simulink model "LPVMPC_AGV_simulink"  (R2024b)
settings: Solver=ode4  StartTime=0.0  StopTime=20  FixedStep=0.05  RelTol=1e-3
PreLoadFcn:
  | %% PreLoadFcn - 自动路径兼容版 V3.0 (2025-12-10)
  | fprintf('\n');
  | fprintf('╔════════════════════════════════════════════════════════════╗\n');
  | fprintf('║     LPVMPC_AGV 模型初始化 (PreLoadFcn, V3.0, 2025-12-10)   ║\n');
  | fprintf('╚════════════════════════════════════════════════════════════╝\n\n');
  | 
  | %% Bootstrap path + 目录配置
  | init_project();
  | root = project_root();
  | data_dir = fullfile(root, 'data');
  | data_models_dir = fullfile(data_dir, 'models');
  | data_paths_dir = fullfile(data_dir, 'paths');
  | data_gru_dir = fullfile(data_dir, 'gru');
  | results_root = results_dir('');
  | results_paths = struct( ...
  |     'root', results_root, ...
  |     'simulink', results_dir('simulink'), ...
  |     'closed_loop', results_dir('closed_loop'), ...
  |     'paths', results_dir('paths'), ...
  |     'gru_logs', results_dir('gru/sim'));
  | env_paths = struct('root', root, 'data', data_dir, 'models', data_models_dir, ...
  |     'paths', data_paths_dir, 'gru', data_gru_dir, 'results', results_paths);
  | 
  | assignin('base', 'results_paths', results_paths);
  | assignin('base', 'env_paths', env_paths);
  | 
  | mw = get_param(bdroot, 'ModelWorkspace');
  | assignin(mw, 'results_paths', results_paths);
  | assignin(mw, 'env_paths', env_paths);
  | try, save(mw); catch, end
  | 
  | %% 步骤0：加载基础参数
  | fprintf('[步骤 0/6] 加载基础参数...\n');
  | try
  |     params = parameters();
  |     fprintf('  ✓ parameters() 加载成功 (Ts=%.3fs, m=%.1fkg, L=%.2fm)\n', ...
  |         params.Ts, params.mass, params.L);
  | catch ME
  |     warning('[PreLoadFcn] parameters() 失败: %s', ME.message);
  |     params = struct('Ts',0.05,'mass',100,'gravity',9.81, ...
  |         'rolling_resistance',0.015,'air_density',1.225, ...
  |         'drag_coefficient_area',0.5,'L',2.0);
  | end
  | assignin('base','params',params);
  | assignin(mw,'params',params);
  | 
  | ff_rt = struct('m',params.mass,'g',params.gravity, ...
  |     'c_r',params.rolling_resistance,'rho',params.air_density, ...
  |     'CdA',params.drag_coefficient_area);
  | v_ff_nom = 1.0;
  | assignin('base','ff_rt',ff_rt);
  | assignin('base','v_ff_nom',v_ff_nom);
  | assignin(mw,'ff_rt',ff_rt);
  | assignin(mw,'v_ff_nom',v_ff_nom);
  | try, save(mw); catch, end
  | fprintf('\n');
  | 
  | %% 步骤1：载入 LPV 数据库
  | fprintf('[步骤 1/6] 加载 LPV 数据库...\n');
  | base_names = {'lin_agv_db.mat','plant_grid_test.mat','plant_grid.mat'};
  | base_dirs = {data_models_dir, root, ''};
  | db_files = {};
  | for d = 1:numel(base_dirs)
  |     for n = 1:numel(base_names)
  |         if isempty(base_dirs{d})
  |             db_files{end+1} = base_names{n}; %#ok<AGROW>
  |         else
  |             db_files{end+1} = fullfile(base_dirs{d}, base_names{n}); %#ok<AGROW>
  |         end
  |     end
  | end
  | db_files = unique(db_files, 'stable');
  | 
  | S = [];
  | loaded_db_file = '';
  | for i = 1:numel(db_files)
  |     if exist(db_files{i}, 'file')
  |         try
  |             S = load(db_files{i});
  |             loaded_db_file = db_files{i};
  |             fprintf('  ✓ 文件加载成功: %s\n', db_files{i});
  |             break;
  |         catch ME
  |             fprintf('  ⚠ 尝试加载 %s 失败: %s\n', db_files{i}, ME.message);
  |         end
  |     end
  | end
  | 
  | if isempty(S)
  |     error('[PreLoadFcn] ❌ 未找到 LPV 数据库文件（请先运行 lin_agv_grid 或 test_lpvmpc_workflow）');
  | end
  | 
  | if isfield(S,'db') && isstruct(S.db)
  |     db_data = S.db;
  |     fprintf('  → 使用 db 结构体格式\n');
  | elseif all(isfield(S, {'A','B','C','D','E'}))
  |     db_data = S;
  |     fprintf('  → 使用顶层字段格式\n');
  | else
  |     error('[PreLoadFcn] 数据库格式无法识别 (字段: %s)', strjoin(fieldnames(S), ', '));
  | end
  | 
  | req = {'A','B','C','D','E','Ts','grid'};
  | missing = req(~isfield(db_data, req));
  | if ~isempty(missing)
  |     error('[PreLoadFcn] ❌ 数据库缺少字段: %s', strjoin(missing, ', '));
  | end
  | 
  | A=db_data.A; B=db_data.B; C=db_data.C; D=db_data.D; E=db_data.E;
  | Ts=db_data.Ts; grid=db_data.grid;
  | nx=size(A,4); nu=size(B,5); ny=size(C,4); nd=size(E,5);
  | Nv=size(A,1); Nw=size(A,2); Nt=size(A,3);
  | 
  | fprintf('  ✓ 网格: %d×%d×%d (总 %d 点), nx=%d, nu=%d, nd=%d, Ts=%.3fs\n', ...
  |     Nv, Nw, Nt, Nv*Nw*Nt, nx, nu, nd, Ts);
  | 
  | db_rt = struct('A',A,'B',B,'C',C,'D',D,'E',E, ...
  |     'grid',grid,'Ts',Ts,'nx',nx,'nu',nu,'ny',ny,'nd',nd, ...
  |     'Nv',Nv,'Nw',Nw,'Nt',Nt);
  | assignin('base','db_rt',db_rt);
  | assignin(mw,'db_rt',db_rt);
  | try, save(mw); catch, end
  | fprintf('\n');
  | 
  | %% 步骤2：创建 MPCPlantBus
  | fprintf('[步骤 2/6] 创建 MPCPlantBus...\n');
  | nu_md = nu + nd;
  | samplePlant = struct('A',zeros(nx,nx),'B',zeros(nx,nu_md), ...
  |     'C',zeros(ny,nx),'D',zeros(ny,nu_md),'U',zeros(nu_md,1), ...
  |     'X',zeros(nx,1),'Y',zeros(ny,1),'DX',zeros(nx,1),'Ts',Ts);
  | info = Simulink.Bus.createObject(samplePlant);
  | assignin('base','MPCPlantBus', eval(info.busName));
  | if ~strcmp(info.busName,'MPCPlantBus')
  |     eval(sprintf('clear %s;', info.busName));
  | end
  | assignin('base','plant_ic', samplePlant);
  | fprintf('  ✓ MPCPlantBus 创建成功 (nu_md=%d = %d MV + %d MD)\n\n', nu_md, nu, nd);
  | 
  | %% 步骤3：加载 maps_best / ctrl
  | fprintf('[步骤 3/6] 加载 maps_best / ctrl...\n');
  | base_dirs_mb = {data_models_dir, root, ''};
  | maps_files = {};
  | for d = 1:numel(base_dirs_mb)
  |     if isempty(base_dirs_mb{d})
  |         maps_files{end+1} = 'maps_best.mat'; %#ok<AGROW>
  |     else
  |         maps_files{end+1} = fullfile(base_dirs_mb{d}, 'maps_best.mat'); %#ok<AGROW>
  |     end
  | end
  | maps_files = unique(maps_files, 'stable');
  | 
  | maps_best = [];
  | maps_loaded = false;
  | for i = 1:numel(maps_files)
  |     if exist(maps_files{i}, 'file')
  |         try
  |             Tm = load(maps_files{i});
  |             if isfield(Tm,'maps_best')
  |                 maps_best = Tm.maps_best;
  |                 maps_loaded = true;
  |                 fprintf('  ✓ maps_best 加载成功 (%s)\n', maps_files{i});
  |                 if isfield(maps_best,'version')
  |                     fprintf('    - 版本: %s\n', maps_best.version);
  |                 end
  |                 if isfield(maps_best,'timestamp')
  |                     fprintf('    - 时间: %s\n', maps_best.timestamp);
  |                 end
  |             end
  |             break;
  |         catch ME
  |             fprintf('  ⚠ 加载 %s 失败: %s\n', maps_files{i}, ME.message);
  |         end
  |     end
  | end
  | if ~maps_loaded
  |     fprintf('  ⚠ 未找到 maps_best.mat，使用默认权重\n');
  | end
  | 
  | ctrl = [];
  | ctrl_source = '未创建';
  | base_dirs_ctrl = {data_models_dir, root};
  | ctrl_files = {};
  | for d = 1:numel(base_dirs_ctrl)
  |     ctrl_files{end+1} = fullfile(base_dirs_ctrl{d}, 'ctrl.mat'); %#ok<AGROW>
  | end
  | ctrl_files = unique(ctrl_files, 'stable');
  | 
  | for i = 1:numel(ctrl_files)
  |     if exist(ctrl_files{i}, 'file')
  |         try
  |             Tc = load(ctrl_files{i});
  |             if isfield(Tc,'ctrl')
  |                 ctrl = Tc.ctrl;
  |                 ctrl_source = ctrl_files{i};
  |                 fprintf('  ✓ 从 %s 加载 ctrl\n', ctrl_source);
  |                 break;
  |             end
  |         catch ME
  |             fprintf('  ⚠ 加载 %s 失败: %s\n', ctrl_files{i}, ME.message);
  |         end
  |     end
  | end
  | 
  | if isempty(ctrl) && exist('mpc_setup_single_interp','file')==2
  |     fprintf('  → 创建新控制器...\n');
  |     if maps_loaded && all(isfield(maps_best, {'Q_range','R_range','dR_range'}))
  |         Q_base = mean(maps_best.Q_range,1);
  |         R_base = mean(maps_best.R_range,1);
  |         dR_base = mean(maps_best.dR_range,1);
  |         fprintf('    使用 maps_best 权重\n');
  |     else
  |         Q_base = [3,8,1,1];
  |         R_base = [1e-3,1e-3];
  |         dR_base = [1e-2,1e-2];
  |         fprintf('    使用默认权重\n');
  |     end
  |     mpc_opts = struct('Np',30,'Nc',10,'Q',Q_base,'R',R_base,'dR',dR_base);
  |     ctrl = mpc_setup_single_interp(db_rt, mpc_opts);
  |     ctrl_source = '新创建';
  |     fprintf('  ✓ 控制器创建成功 (P=%.2fs, M=%.2fs)\n', ...
  |         ctrl.meta.prediction_horizon_sec, ctrl.meta.control_horizon_sec);
  | end
  | 
  | if maps_loaded && ~isempty(ctrl)
  |     fields = {'Q_range','R_range','dR_range','alpha_Q','beta_Q', ...
  |         'alpha_R','beta_R','alpha_dR','beta_dR', ...
  |         'scale_umin_lo','scale_umin_hi','scale_umax_lo','scale_umax_hi'};
  |     copied = 0;
  |     for i = 1:numel(fields)
  |         if isfield(maps_best, fields{i})
  |             ctrl.maps.(fields{i}) = maps_best.(fields{i});
  |             copied = copied + 1;
  |         end
  |     end
  |     fprintf('  → 已将 %d 个 maps_best 字段写入 ctrl.maps\n', copied);
  | end
  | 
  | if ~isempty(ctrl)
  |     assignin('base','ctrl',ctrl);
  | else
  |     warning('[PreLoadFcn] 无法创建/加载 ctrl');
  | end
  | fprintf('\n');
  | 
  | %% 步骤4：直接加载参考路径到基础工作区
  | % fprintf('[步骤 4/6] 加载路径参考数据（ref_* 格式）...\n');
  | %
  | % path_types = {'straight','turn','straight_left_turn','straight_right_turn','slope','bumpy', ...
  | %               's_curve','s_shape'};
  | % path_refs = struct();
  | % paths_loaded = 0;
  | %
  | % for i = 1:numel(path_types)
  | %     name = path_types{i};
  | %     file_path = fullfile(data_paths_dir, sprintf('path_%s.mat', name));
  | %     if ~exist(file_path,'file')
  | %         fprintf('  ⚠ 缺少路径文件: %s\n', file_path);
  | %         continue;
  | %     end
  | %
  | %     try
  | %         data = load(file_path);
  | %         if ~isfield(data,'ref')
  | %             error('文件缺少 ref 结构');
  | %         end
  | %         ref = data.ref;
  | %         var_name = sprintf('ref_%s', name);
  | %
  | %         % 写入 Base Workspace（兼容旧流程）
  | %         assignin('base', var_name, ref);
  | %         % 如需模型工作区可同步写入
  | %         assignin(mw, var_name, ref);
  | %
  | %         % 记录到 path_refs 结构
  | %         path_refs.(name) = ref;
  | %
  | %         paths_loaded = paths_loaded + 1;
  | %         fprintf('  ✓ %s: 已加载 (%s → %s)\n', name, file_path, var_name);
  | %     catch ME
  | %         fprintf('  ❌ 加载 %s 失败: %s\n', name, ME.message);
  | %     end
  | % end
  | %
  | % assignin('base','path_refs',path_refs);
  | % assignin(mw,'path_refs',path_refs);
  | % try, save(mw); catch, end
  | % fprintf('  → 路径数据加载 %d/%d\n\n', paths_loaded, numel(path_types));
  | %% 步骤5：加载 GRU 模型
  | fprintf('[步骤 5/6] 加载 GRU 模型...\n');
  | gru_model = [];
  | gru_scaler = [];
  | 
  | base_dirs_gru = {data_models_dir, data_gru_dir, root};
  | gru_files = {};
  | for d = 1:numel(base_dirs_gru)
  |     gru_files{end+1} = fullfile(base_dirs_gru{d}, 'GRU_model.mat'); %#ok<AGROW>
  | end
  | gru_files = unique(gru_files, 'stable');
  | 
  | for i = 1:numel(gru_files)
  |     if exist(gru_files{i},'file')
  |         Sg = load(gru_files{i});
  |         if isfield(Sg,'model')
  |             gru_model = Sg.model;
  |             fprintf('  ✓ GRU_model 加载成功 (%s)\n', gru_files{i});
  |             if isfield(gru_model,'seq_len')
  |                 fprintf('    - 序列长度: %d\n', gru_model.seq_len);
  |             end
  |             if isfield(gru_model,'scaler')
  |                 gru_scaler = gru_model.scaler;
  |             end
  |             break;
  |         end
  |     end
  | end
  | if isempty(gru_model)
  |     error('[PreLoadFcn] ❌ 未找到 GRU_model.mat');
  | end
  | 
  | scaler_files = {};
  | for d = 1:numel(base_dirs_gru)
  |     scaler_files{end+1} = fullfile(base_dirs_gru{d}, 'GRU_scaler.mat'); %#ok<AGROW>
  | end
  | scaler_files = unique(scaler_files, 'stable');
  | if isempty(gru_scaler)
  |     for i = 1:numel(scaler_files)
  |         if exist(scaler_files{i},'file')
  |             Ss = load(scaler_files{i});
  |             if isfield(Ss,'scaler')
  |                 gru_scaler = Ss.scaler;
  |                 fprintf('  ✓ GRU_scaler 加载成功 (%s)\n', scaler_files{i});
  |                 break;
  |             end
  |         end
  |     end
  | end
  | 
  | assignin('base','gru_model',gru_model);
  | if ~isempty(gru_scaler)
  |     assignin('base','gru_scaler',gru_scaler);
  | end
  | fprintf('\n');
  | 
  | %% 步骤6：总结
  | fprintf('[步骤 6/6] 初始化总结\n');
  | fprintf('  ════════════════════════════════════════════════\n');
  | fprintf('  ✓ 基础参数:     已加载\n');
  | fprintf('  ✓ LPV 数据库:   %s (%d×%d×%d)\n', loaded_db_file, Nv, Nw, Nt);
  | fprintf('  ✓ MPCPlantBus:  已创建\n');
  | % fprintf('  ✓ 路径数据:     %d/%d\n', paths_loaded, numel(path_types));
  | fprintf('  ✓ GRU 模型:     就绪\n');
  | if maps_loaded
  |     fprintf('  ✓ maps_best:    已加载\n');
  | else
  |     fprintf('  ⚠ maps_best:    未加载\n');
  | end
  | if ~isempty(ctrl)
  |     fprintf('  ✓ MPC 控制器:   %s\n', ctrl_source);
  | else
  |     fprintf('  ❌ MPC 控制器:  未创建\n');
  | end
  | fprintf('  ════════════════════════════════════════════════\n');
  | 
  | if maps_loaded && ~isempty(ctrl)
  |     fprintf('\n✓ 初始化成功！使用优化权重与 GRU 调度\n');
  | elseif ~isempty(ctrl)
  |     fprintf('\n⚠ 初始化完成，使用默认权重\n');
  | else
  |     fprintf('\n❌ 初始化失败，请检查上方日志\n');
  | end
  | fprintf('\n[PreLoadFcn] 完成\n\n');
model workspace (MAT data in the model file):
  CdA = 0.5
  MPC_idx = [1 2 3 4]
  c_r = 0.015
  db_rt.A = [1 1 1 1 1 1 1 1 1 1 1 1 ... (2000 elements, 5x5x5x4x4)]
  db_rt.B = [1.10696819051e-09 6.56859347141e-11 7.70788358052e-11 4.63456222969e-11 -1.91478442817e-11 3.08062125377e-10 3.17967815903e-10 3.27251111689e-10 3.36091973111e-10 3.44604983367e-10 -2.40695313568e-13 -1.34215112609e-13 ... (1000 elements, 5x5x5x4x2)]
  db_rt.C = [1 1 1 1 1 1 1 1 1 1 1 1 ... (2000 elements, 5x5x5x4x4)]
  db_rt.D = [0 0 0 0 0 0 0 0 0 0 0 0 ... (1000 elements, 5x5x5x4x2)]
  db_rt.E = [2.11033585519e-07 -6.42122832244e-08 -7.53495772598e-08 -4.53058513965e-08 1.871832239e-08 -3.01151562194e-07 -3.10835010863e-07 -3.19910021986e-07 -3.2855251907e-07 -3.36874515032e-07 2.35296065713e-10 1.31204413144e-10 ... (500 elements, 5x5x5x4)]
  db_rt.grid.V = [0.8; 0.9; 1; 1.1; 1.2]
  db_rt.grid.W = [-0.2; -0.1; 0; 0.1; 0.2]
  db_rt.grid.T = [-0.1; -0.05; 0; 0.05; 0.1]
  db_rt.Ts = 0.01
  db_rt.nx = 4
  db_rt.nu = 2
  db_rt.ny = 4
  db_rt.nd = 1
  db_rt.Nv = 5
  db_rt.Nw = 5
  db_rt.Nt = 5
  g = 9.81
  m = 100
  rho = 1.225
libraries: mpclib x1
settings Model: Creator=15754  LastModifiedBy=15754

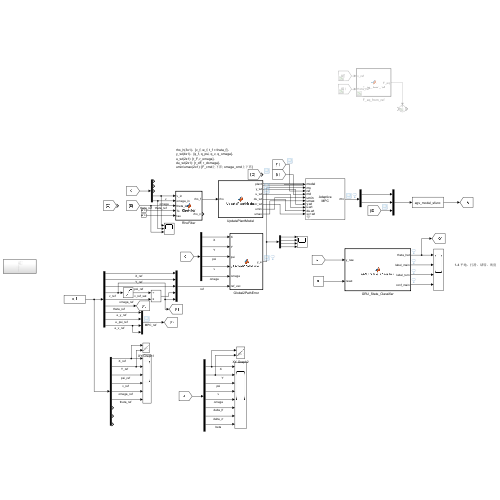
[thumbnail: Simulink's stored preview of the top-level diagram]
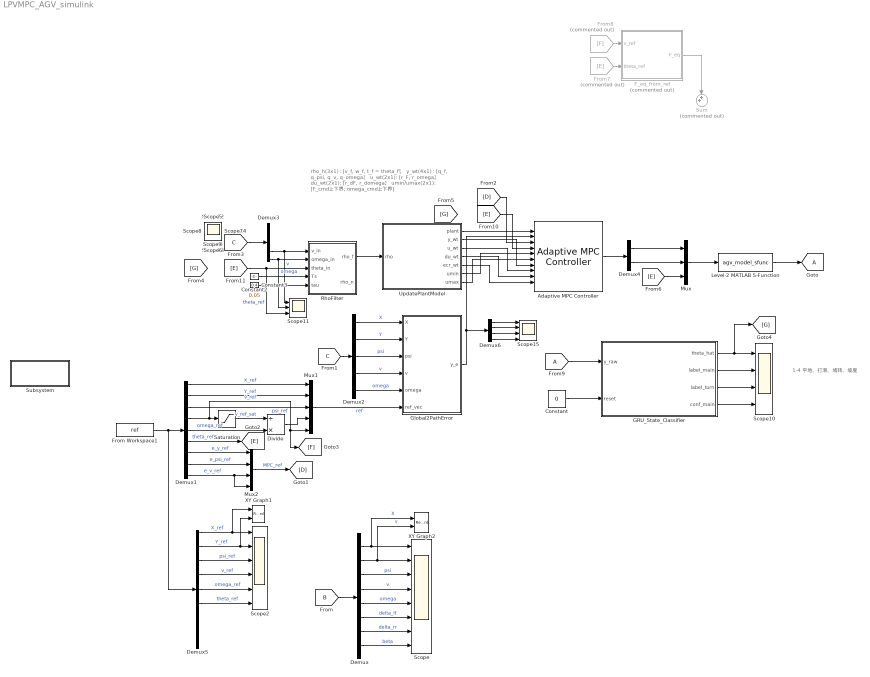
== system LPVMPC_AGV_simulink ==
  note: rho_h(3x1)：[v_f, w_f, t_f = theta_f]。
      | y_wt(4x1)：[q_f, q_psi, q_v, q_omega]。
      | u_wt(2x1): [r_F, r_omega]。
      | du_wt(2x1): [r_dF, r_domega]。
      | umin/umax(2x1): [F_cmd上下界; omega_cmd上下界]
  note: 1-4 平地、打滑、堵转、坡度
  Adaptive MPC Controller : mpclib/Adaptive MPC Controller  SCDEnableBlockLinearizationSpecification=on  mpcobj=ctrl.mpcobj  enable_value=0  updateMPCinCallerWorkspace=on  md_inport=on  mv_inport=off  uref_inport=off  return_cost=off  return_mvseq=off  return_qpstatus=off  return_xseq=off  return_state=off  return_ovseq=off  state_inport=off  isltv_plant=off  umin_inport=on  umax_inport=on  ymin_inport=off  ymax_inport=off  cc_inport=off  ywt_inport=on  uwt_inport=on  duwt_inport=on  rhoeps_inport=on  pm_inport=off  MaximumP=10  HorizonChoice=FixedHorizon  BlockDataType=double  SampleTimeInherited=off  switch_inport=off
  Constant : Constant  Value=0  SampleTime=params.Ts
  Constant2 : Constant  Value=0.05  SampleTime=params.Ts
  Constant3 : Constant  Value=0.4  SampleTime=params.Ts
  Demux : Demux  Outputs=8
  Demux1 : Demux  Outputs=9
  Demux2 : Demux  Outputs=5
  Demux3 : Demux  Outputs=5
  Demux4 : Demux  Outputs=2
  Demux5 : Demux  Outputs=9
  Demux6 : Demux
  Divide : Product  Inputs=/*
  F_eq_from_ref : MATLAB Function  Commented=on  TreatAsAtomicUnit=on
  From Workspace1 : FromWorkspace  VariableName=ref  SampleTime=0.05
  From7 : From  Commented=on  GotoTag=E
  From8 : From  Commented=on  GotoTag=F
  From9 : From  TagVisibility=global
  GRU_State_Classifier : MATLAB Function  TreatAsAtomicUnit=on
  Global2PathError : MATLAB Function  TreatAsAtomicUnit=on  SystemSampleTime=params.Ts
  Goto : Goto  TagVisibility=global
  Level-2 MATLAB S-Function : M-S-Function  FunctionName=agv_model_sfunc  Parameters=parameters
  Mux : Mux  Inputs=3
  Mux1 : Mux  Inputs=5
  Mux2 : Mux
  RhoFilter : MATLAB Function  TreatAsAtomicUnit=on  SystemSampleTime=0.05
  Saturation : Saturate  UpperLimit=Inf  LowerLimit=1e-3
  Scope : Scope  NumInputPorts=8
  Scope10 : Scope  NumInputPorts=4
  Scope11 : Scope  NumInputPorts=3
  Scope15 : Scope  NumInputPorts=4
  Scope2 : Scope  NumInputPorts=6
  Subsystem : Subsystem
  Sum : Sum  Commented=on  Inputs=++|
  UpdatePlantModel : MATLAB Function  TreatAsAtomicUnit=on
  XY Graph1 : Record  FileSettingsInternal="{\"entries\":[{\"content\":{\"excelSettings\":{\"content\":{},\"type\":\"Streamout.ExcelSettings\"}},\"type\":\"Streamout.FileSettingStorage\",\"uuid\":\"\"}],\"packageUris\":[\"http:\\/\\/schema.mathworks.com\\/mf0\\/streamout_blocks\\/R2020a\"],\"version\":\"1.0\"}"  Layout=[1 1]  SignalsInternal="{\"entries\":[{\"content\":{\"signals\":[{\"content\":{\"blockPath\":[],\"dimensions\":[1],\"domain\":\"\",\"lineColor\":\"#a2142f\",\"plots\":[ 1 ],\"port\":1,\"sid\":[\"\"],\"signalID\":1,\"signalName\":\"X_ref\"},\"type\":\"RecordBlkView.Signal\",\"uuid\":\"\"},{\"content\":{\"blockPath\":[],\"dimensions\":[1],\"domain\":\"\",\"lineColor\":\"#139fff\",\"plots\":[ 1 ],\"port\":2,\"sid\":[\"\"],\"signalID\":2,\"signalName\":\"Y_ref\"},\"type\":\"RecordBlkView.Signal\",\"uuid\":\"\"}]},\"type\":\"RecordBlkView.InputSignals\",\"uuid\":\"\"}],\"packageUris\":[\"http:\\/\\/schema.mathworks.com\\/mf0\\/streamout_blocks\\/R2020a\"],\"version\":\"1.0\"}"  VisualizationBindings="{\"xyplotplugin\":{\"info\":[{\"series\":[{\"bindingParametersList\":[{\"parameter\":\"X-Axis\",\"signalID\":1,\"signalName\":\"X_ref\"},{\"parameter\":\"Y-Axis\",\"signalID\":2,\"signalName\":\"Y_ref\"}],\"seriesID\":0}],\"subplotID\":1}]}}"  CompatibilityTag=XY
  XY Graph2 : Record  FileSettingsInternal="{\"entries\":[{\"content\":{\"excelSettings\":{\"content\":{},\"type\":\"Streamout.ExcelSettings\"}},\"type\":\"Streamout.FileSettingStorage\",\"uuid\":\"\"}],\"packageUris\":[\"http:\\/\\/schema.mathworks.com\\/mf0\\/streamout_blocks\\/R2020a\"],\"version\":\"1.0\"}"  Layout=[1 1]  SignalsInternal="{\"entries\":[{\"content\":{\"signals\":[{\"content\":{\"blockPath\":[],\"dimensions\":[1],\"domain\":\"\",\"lineColor\":\"#a2142f\",\"plots\":[ 1 ],\"port\":1,\"sid\":[\"\"],\"signalID\":1,\"signalName\":\"X\"},\"type\":\"RecordBlkView.Signal\",\"uuid\":\"\"},{\"content\":{\"blockPath\":[],\"dimensions\":[1],\"domain\":\"\",\"lineColor\":\"#139fff\",\"plots\":[ 1 ],\"port\":2,\"sid\":[\"\"],\"signalID\":2,\"signalName\":\"Y\"},\"type\":\"RecordBlkView.Signal\",\"uuid\":\"\"}]},\"type\":\"RecordBlkView.InputSignals\",\"uuid\":\"\"}],\"packageUris\":[\"http:\\/\\/schema.mathworks.com\\/mf0\\/streamout_blocks\\/R2020a\"],\"version\":\"1.0\"}"  VisualizationBindings="{\"xyplotplugin\":{\"info\":[{\"series\":[{\"bindingParametersList\":[{\"parameter\":\"X-Axis\",\"signalID\":1,\"signalName\":\"X\"},{\"parameter\":\"Y-Axis\",\"signalID\":2,\"signalName\":\"Y\"}],\"seriesID\":0}],\"subplotID\":1}]}}"  CompatibilityTag=XY
  Scope{1,3..9,12..14} (11 alike) : Scope
  wires:
  Level-2 MATLAB S-Function/1 -> Goto/1
  [B] -> Demux/1
  Demux/1 -> XY Graph2/1, Scope/1  "X"
  Demux/2 -> XY Graph2/2, Scope/2  "Y"
  Demux/3 -> Scope/3  "psi"
  Demux/4 -> Scope/4  "v"
  Demux/5 -> Scope/5  "omega"
  Demux/6 -> Scope/6  "delta_lf"
  Demux/7 -> Scope/7  "delta_rr"
  Demux/8 -> Scope/8  "beta"
  Demux1/4 -> [F], Mux1/5, Saturation/1  "v_ref"
  Saturation/1 -> Divide/1  "v_ref_sat"
  Demux1/5 -> Divide/2  "omega_ref"
  Demux1/1 -> Mux1/1  "X_ref"
  Demux1/2 -> Mux1/2  "Y_ref"
  Demux1/3 -> Mux1/3  "psi_ref"
  Divide/1 -> Mux1/4
  Mux1/1 -> Global2PathError/6(ref_vec)  "ref"
  [C] -> Demux2/1
  Demux2/3 -> Global2PathError/3(psi)  "psi"
  Demux2/4 -> Global2PathError/4(v)  "v"
  Demux2/5 -> Global2PathError/5(omega)  "omega"
  Demux2/2 -> Global2PathError/2(Y)  "Y"
  Demux2/1 -> Global2PathError/1(X)  "X"
  Demux1/8 -> Mux2/2  "e_psi_ref"
  Demux1/7 -> Mux2/1  "e_y_ref"
  Demux1/9 -> Mux2/4, Mux2/3  "e_v_ref"
  Mux2/1 -> [D]  "MPC_ref"
  [D] -> Adaptive MPC Controller/3
  [C] -> Demux3/1
  Demux3/4 -> Scope11/1, RhoFilter/1(v_in)  "v"
  Demux3/5 -> Scope11/2, RhoFilter/2(omega_in)  "omega"
  Demux1/6 -> [E]  "theta_ref"
  [E] -> Scope11/3, RhoFilter/3(theta_in)  "theta_ref"
  Constant2/1 -> RhoFilter/4(Ts)
  Constant3/1 -> RhoFilter/5(tau)
  UpdatePlantModel/1(plant) -> Adaptive MPC Controller/1
  [E] -> Adaptive MPC Controller/4
  RhoFilter/1(rho_f) -> UpdatePlantModel/1(rho)
  Demux5/1 -> XY Graph1/1, Scope2/1  "X_ref"
  Demux5/2 -> XY Graph1/2, Scope2/2  "Y_ref"
  Demux5/3 -> Scope2/3  "psi_ref"
  Demux5/4 -> Scope2/4  "v_ref"
  Demux5/5 -> Scope2/5  "omega_ref"
  Demux5/6 -> Scope2/6  "theta_ref"
  UpdatePlantModel/6(umin) -> Adaptive MPC Controller/5
  UpdatePlantModel/7(umax) -> Adaptive MPC Controller/6
  UpdatePlantModel/2(y_wt) -> Adaptive MPC Controller/7
  UpdatePlantModel/3(u_wt) -> Adaptive MPC Controller/8
  UpdatePlantModel/4(du_wt) -> Adaptive MPC Controller/9
  UpdatePlantModel/5(ecr_wt) -> Adaptive MPC Controller/10
  Global2PathError/1(y_e) -> Demux6/1, Adaptive MPC Controller/2
  Mux/1 -> Level-2 MATLAB S-Function/1
  Adaptive MPC Controller/1 -> Demux4/1
  [E] -> Mux/3
  Demux4/2 -> Mux/2
  F_eq_from_ref/1(F_eq) -> Sum/1
  From8/1 -> F_eq_from_ref/1(v_ref)
  From7/1 -> F_eq_from_ref/2(theta_ref)
  Demux4/1 -> Mux/1
  From9/1 -> GRU_State_Classifier/1(y_raw)
  GRU_State_Classifier/4(conf_main) -> Scope10/4
  GRU_State_Classifier/2(label_main) -> Scope10/2
  Constant/1 -> GRU_State_Classifier/2(reset)
  GRU_State_Classifier/3(label_turn) -> Scope10/3
  GRU_State_Classifier/1(theta_hat) -> [G], Scope10/1
  From Workspace1/1 -> Demux5/1, Demux1/1
  Demux6/1 -> Scope15/1
  Demux6/2 -> Scope15/2
  Demux6/3 -> Scope15/3
  Demux6/4 -> Scope15/4

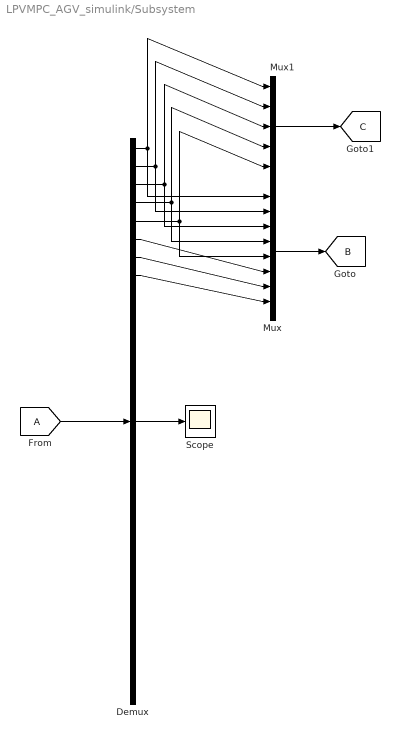
== system LPVMPC_AGV_simulink/Subsystem ==
  Demux : Demux  Outputs=31
  From : From  TagVisibility=global
  Mux : Mux  Inputs=8
  Mux1 : Mux  Inputs=5
  Scope : Scope
  tag scope: B=global, C=global
  wires:
  From/1 -> Demux/1
  Demux/1 -> Mux1/1, Mux/1
  Demux/2 -> Mux1/2, Mux/2
  Demux/3 -> Mux1/3, Mux/3
  Demux/4 -> Mux1/4, Mux/4
  Demux/5 -> Mux1/5, Mux/5
  Demux/6 -> Mux/6
  Demux/7 -> Mux/7
  Demux/8 -> Mux/8
  Mux/1 -> [B]
  Mux1/1 -> [C]
  Demux/16 -> Scope/1

== matlab function LPVMPC_AGV_simulink/RhoFilter ==
  data: v_in input; rho_f output; omega_in input; theta_in input; Ts input; tau input; rho_n output
function [rho_f, rho_n] = RhoFilter(v_in, omega_in, theta_in, Ts, tau)
% 一阶离散滤波
persistent v_f_prev w_f_prev t_f_prev
if isempty(v_f_prev), v_f_prev = 0; end
if isempty(w_f_prev), w_f_prev = 0; end
if isempty(t_f_prev), t_f_prev = 0; end

a = Ts / max(tau + Ts, 1e-6);

v_f = (1 - a)*v_f_prev + a*max(v_in, 0);   % 速度不取负·
w_f = (1 - a)*w_f_prev + a*omega_in;       % 保留符号
t_f = (1 - a)*t_f_prev + a*theta_in;       % 保留符号

v_f_prev = v_f; w_f_prev = w_f; t_f_prev = t_f;

rho_f = [v_f; w_f; t_f];

% 可选归一化（仅用于监控/调试，不参与UpdatePlantModel）
Vmax = 2.0; Wmax = 0.8; Tmax = deg2rad(10);
rho_n = [min(v_f/Vmax,1); min(abs(w_f)/Wmax,1); min(abs(t_f)/Tmax,1)];
end

== matlab function LPVMPC_AGV_simulink/Global2PathError ==
  data: X input; y_e output; Y input; psi input; v input; omega input; ref_vec input
% 误差计算模块
function y_e = Global2PathError(X, Y, psi, v, omega, ref_vec)
% ref_vec = [X_ref; Y_ref; psi_ref; kappa_ref; v_ref]
% 输出: y_e = [e_y; e_psi; e_v; e_omega; e_s]

%#codegen
% 1) 解包参考
Xr = ref_vec(1);
Yr = ref_vec(2);
psir = ref_vec(3);
kappa = ref_vec(4);
v_ref = ref_vec(5);

% 2) 横向误差：沿参考法向量投影（带符号）
ex = X - Xr; 
ey = Y - Yr;
e_y = -sin(psir)*ex + cos(psir)*ey;

% 3) 航向、速度、角速度误差
e_psi   = wrapToPi(psi - psir);
e_v     = v - v_ref;
omega_ff= v_ref * kappa;           % 曲率前馈
e_omega = omega - omega_ff;

% 4) 进度误差（可选，如未使用可置 0）
e_s = 0;

y_e = [e_y; e_psi; e_v; e_omega];
end

== matlab function LPVMPC_AGV_simulink/UpdatePlantModel ==
  data: rho input; plant output Bus: MPCPlantBus; db_rt parameter; MPC_idx parameter double size=[1 4]; ff_rt parameter; v_ff_nom parameter; y_wt output; u_wt output; du_wt output; ecr_wt output; umin output; umax output
function [plant, y_wt, u_wt, du_wt, ecr_wt, umin, umax] = UpdatePlantModel(rho, db_rt, MPC_idx, ff_rt, v_ff_nom)
%#codegen

% 标称权重/约束
Q0  = [16.3225, 29.0359, 6.9898, 2.7642];
% Q0  = [3, 8, 1, 1];
R0  = [1e-3, 1e-3];
dR0 = [1e-2, 1e-2];
umin0 = [-300; -0.6];
umax0 = [ 300;  0.6];

% 纯数值 maps：启用 ρ→(Q/R/dR/umin/umax)
maps_local = struct();
maps_local.enable_weight_interp = true;
maps_local.Q_range  = [0.5*Q0; 1.5*Q0];
maps_local.R_range  = [0.5*R0; 1.5*R0];
maps_local.dR_range = [0.5*dR0; 1.5*dR0];
% 约束：随 |ω| 插值（行1→行2）
maps_local.umin_range = [ (1.20*umin0).'; (1.00*umin0).' ];
maps_local.umax_range = [ (1.00*umax0).'; (1.20*umax0).' ];

% 在线插值
upd = mpc_update_from_rho(rho, db_rt, maps_local);

% 组装 3 输入（2 MV + 1 MD）
A   = upd.A; Bmv = upd.B; C = upd.C; Dmv = upd.D;
nx  = size(A,1); ny = size(C,1); nd = 1;
if isfield(upd,'E') && ~isempty(upd.E), Bmd = upd.E(:,1); else, Bmd = zeros(nx,1); end
Dmd = zeros(ny,nd);

plant.A = A;
plant.B = [Bmv, Bmd];   % 4x3
plant.C = C;
plant.D = [Dmv, Dmd];   % 4x3

% 名义 U（仅滚阻+风阻；坡度由 MD 处理）
% theta = rho(3);
% F_rolling = ff_rt.c_r * ff_rt.m * ff_rt.g * cos(theta);
% F_aero    = 0.5 * ff_rt.rho * ff_rt.CdA * v_ff_nom^2;
% F_eq      = F_rolling + F_aero;
% plant.U  = [F_eq; 0; 0];
plant.U  = [0; 0; 0];

% 其它名义量与采样时间（严格按总序）
plant.X  = zeros(nx,1);
plant.Y  = zeros(ny,1);
plant.DX = zeros(nx,1);
plant.Ts = db_rt.Ts;

% 外部权重/约束端口（列向量）
if isfield(upd,'Q') && ~isempty(upd.Q),  y_wt  = upd.Q(:);  else, y_wt  = Q0(:);  end
if isfield(upd,'R') && ~isempty(upd.R),  u_wt  = upd.R(:);  else, u_wt  = R0(:);  end
if isfield(upd,'dR')&& ~isempty(upd.dR), du_wt = upd.dR(:); else, du_wt = dR0(:); end
ecr_wt = 1e4;  % 若需随ρ调度，可按 upd.rho_n 构造插值

if isfield(upd,'umin') && ~isempty(upd.umin), umin = upd.umin(:); else, umin = umin0; end
if isfield(upd,'umax') && ~isempty(upd.umax), umax = upd.umax(:); else, umax = umax0; end
end

== matlab function LPVMPC_AGV_simulink/F_eq_from_ref ==
  data: v_ref input; F_eq output; theta_ref input; m parameter double; g parameter double; c_r parameter double; rho parameter double; CdA parameter double
function F_eq = F_eq_from_ref(v_ref, theta_ref, m, g, c_r, rho, CdA)
%#codegen
% v_ref, theta_ref: 输入端口
% m,g,c_r,rho,CdA  : 本块的 Parameter（标量 double）
v = max(v_ref, 0);
F_roll = c_r * m * g * cos(theta_ref);
F_aero = 0.5 * rho * CdA .* (v.^2);
F_eq = F_roll + F_aero;

% 保持“前馈不含 m·g·sinθ”，以免与 MD 通道重复补偿。

== matlab function LPVMPC_AGV_simulink/GRU_State_Classifier ==
  data theta_hat settings: description=坡度角估计 (rad)
  data label_main settings: description=主分类 [1,2,3,4]
  data label_turn settings: description=转弯状态 [-1, 0, 1]
  data conf_main settings: description=主分类置信度 [0, 1]
  data: y_raw input double size=[31 1]; theta_hat output double size=[1 1]; reset input double size=[1 1]; label_main output double size=[1 1]; label_turn output double size=[1 1]; conf_main output double size=[1 1]
function [theta_hat, label_main, label_turn, conf_main] = GRU_State_Classifier(y_raw, reset)
%#codegen

% ========== 1. 声明 extrinsic 函数 ==========
coder.extrinsic('evalin');
coder.extrinsic('assignin');
coder.extrinsic('GRU_state_classifier');

% ========== 2. 持久变量 ==========
persistent state is_initialized

% ========== 3. 显式初始化输出 ==========
theta_hat = 0.0;
label_main = 1.0;
label_turn = 0.0;
conf_main = 1.0;

% ========== 4. 初始化 ==========
if isempty(is_initialized)
    is_initialized = false;
end

if ~is_initialized || reset == 1
    model = evalin('base', 'gru_model');
    params = evalin('base', 'params');
    state = GRU_state_classifier('init', params, model);
    is_initialized = true;
    return;
end

% ========== 5. 安全检查 ==========
if isempty(state)
    return;
end

% ========== 6. 在线更新 ==========
[state, out] = GRU_state_classifier('update', state, y_raw);

% ========== 7. 提取输出（无需外部文件）==========
assignin('base', 'gru_out_temp', out);
theta_hat = evalin('base', 'double(gru_out_temp.theta_hat)');
label_main = evalin('base', 'double(gru_out_temp.label_main)');
label_turn = evalin('base', 'double(gru_out_temp.label_turn)');
conf_main = evalin('base', 'double(gru_out_temp.conf_main(1))');

end
